simulink model "PickLead_Test_Template"  (R2022b)
settings: Solver=VariableStepAuto  StartTime=0.0  StopTime=50  RelTol=1e-3  EnableMultiTasking=on
libraries: simulink x1
settings Model: Creator=raoulkumar  LastModifiedBy=ryshaw
settings SolverCC: AlgebraicLoopSolver=TrustRegion
settings DataIOCC: LimitDataPoints=on  ReturnWorkspaceOutputs=off
settings OptimizationCC: LifeSpan=inf
settings DebuggingCC: UnconnectedInputMsg=warning  UnconnectedOutputMsg=warning  UnconnectedLineMsg=warning  AllowSymbolicDim=off  SFUnexpectedBacktrackingDiag=warning  SFNoUnconditionalDefaultTransitionDiag=warning  SFExecutionAtInitializationDiag=none  SFMachineParentedDataDiag=warning  ArithmeticOperatorsInVariantConditions=warning
settings ModelReferenceCC: EnableRefExpFcnMdlSchedulingChecks=on  PropagateSignalLabelsOutOfModel=off
settings SFSimCC: SimUseLocalCustomCode=off  CustomCodeUndefinedFunction=UseInterfaceOnly
settings RTWCC: RTWUseLocalCustomCode=off
settings CodeAppCC: StateflowObjectComments=on
settings GRTTargetCC: TargetLangStandard=C89/C90 (ANSI)
settings ConfigComp: CovMetricSettings=dw  CovSaveCumulativeToWorkspaceVar=on  CovSaveSingleToWorkspaceVar=on  CovExternalEMLEnable=off

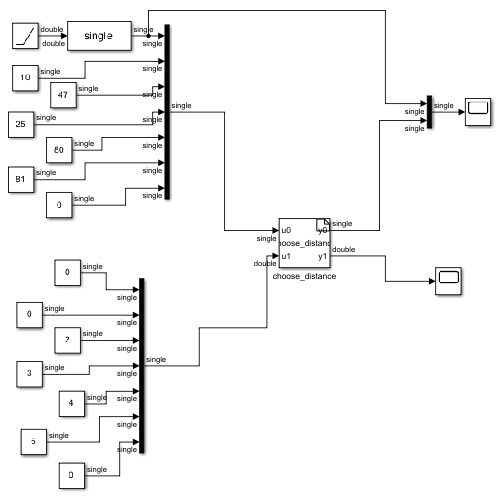
[thumbnail: Simulink's stored preview of the top-level diagram]
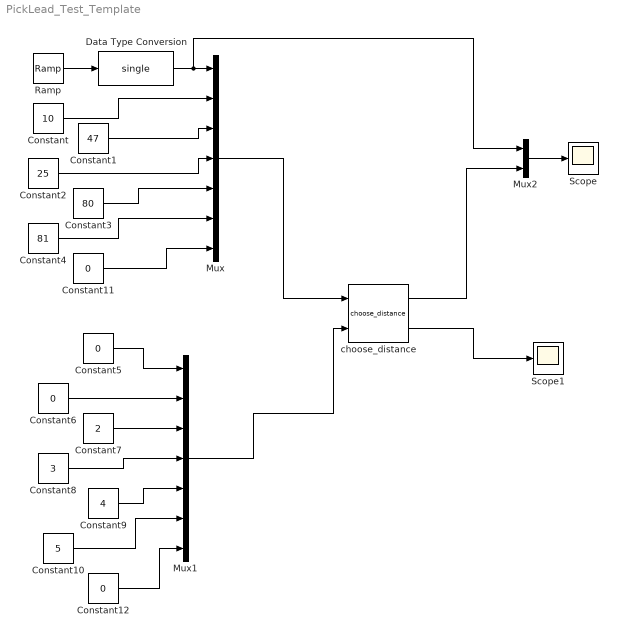
== system PickLead_Test_Template ==
  Constant : Constant  Value=10  OutDataTypeStr=single
  Constant1 : Constant  Value=47  OutDataTypeStr=single
  Constant10 : Constant  Value=5  OutDataTypeStr=single
  Constant{5..6,11..12} (4 alike) : Constant  Value=0  OutDataTypeStr=single
  Constant2 : Constant  Value=25  OutDataTypeStr=single
  Constant3 : Constant  Value=80  OutDataTypeStr=single
  Constant4 : Constant  Value=81  OutDataTypeStr=single
  Constant7 : Constant  Value=2  OutDataTypeStr=single
  Constant8 : Constant  Value=3  OutDataTypeStr=single
  Constant9 : Constant  Value=4  OutDataTypeStr=single
  Data Type Conversion : DataTypeConversion  OutDataTypeStr=single  SaturateOnIntegerOverflow=off  RndMeth=Floor
  Mux : Mux  Inputs=7
  Mux1 : Mux  Inputs=7
  Mux2 : Mux  Inputs=2
  Ramp : simulink/Sources/Ramp  slope=2  start=0  InitialOutput=0
  Scope : Scope
  Scope1 : Scope
  choose_distance : S-Function  FunctionName=choose_distance  SFunctionModules=choose_distance_wrapper.c  SFunctionDeploymentMode=off  EnableBusSupport=off  mask(S-Function Builder){}
      mask help: Simulink:masks:SFunctionBuilder_MD
      mask init:
      | val = [[.9  0.75 0.75 1 1 .9 .9 1]',[1 1 0.75 0.75 .9 .9 1 .9]'];try , sys = get_param(gcb,'SfunBuilderFcnName');if isempty(sys), sys = get_param(gcb,'FunctionName'); end,catch, sys = get_param(gcb,'FunctionName'); end
      settings: CopyFcn=set_param(gcbh,'LinkStatus','none')  OpenFcn=sfunctionwizard(gcbh)
      mask Display:
      | plot(val(:,1),val(:,2))
      | disp(sys)
      | port_label('input',1,'u0')
      | port_label('input',2,'u1')
      | port_label('output',1,'y0')
      | port_label('output',2,'y1')
  wires:
  Mux2/1 -> Scope/1
  Constant/1 -> Mux/2
  Constant1/1 -> Mux/3
  Constant2/1 -> Mux/4
  Constant3/1 -> Mux/5
  Constant4/1 -> Mux/6
  Constant5/1 -> Mux1/1
  Constant6/1 -> Mux1/2
  Constant7/1 -> Mux1/3
  Constant8/1 -> Mux1/4
  Constant9/1 -> Mux1/5
  Constant10/1 -> Mux1/6
  Ramp/1 -> Data Type Conversion/1
  Data Type Conversion/1 -> Mux/1, Mux2/1
  Mux1/1 -> choose_distance/2
  choose_distance/2 -> Scope1/1
  choose_distance/1 -> Mux2/2
  Constant11/1 -> Mux/7
  Constant12/1 -> Mux1/7
  Mux/1 -> choose_distance/1
